simulink model "sampleModel1733_sub_sub"  (R2023a)
settings: Solver=VariableStepAuto  StartTime=0.0  StopTime=10.0  RelTol=1e-3
libraries: hdlsllib x4, simulink x1
settings Model: Creator=user1  LastModifiedBy=user1

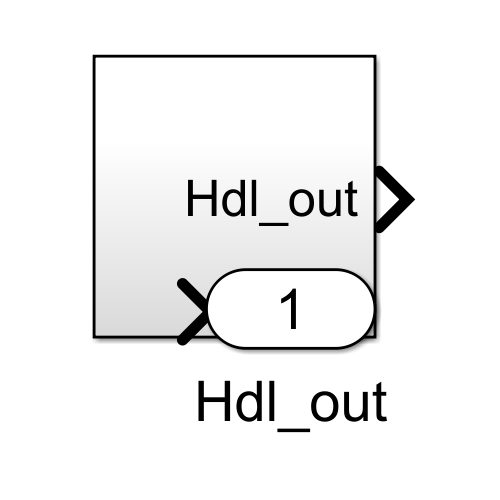
[thumbnail: Simulink's stored preview of the top-level diagram]
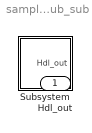
== system sampleModel1733_sub_sub ==
  Subsystem : Subsystem
  Hdl_out : Outport  OutDataTypeStr=uint8

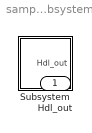
== system sampleModel1733_sub_sub/Subsystem ==
  Subsystem : Subsystem
  Hdl_out : Outport  OutDataTypeStr=uint8

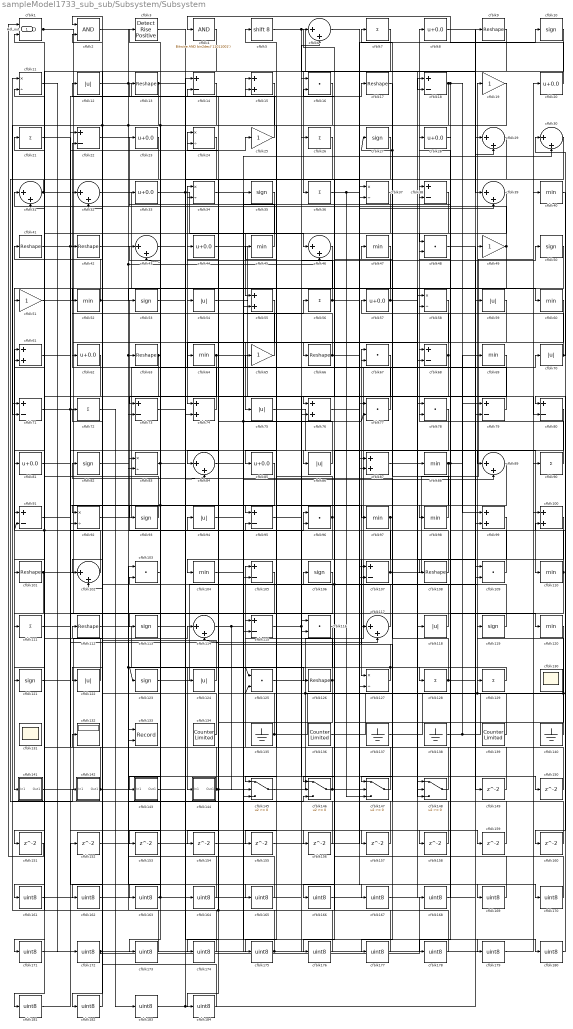
== system sampleModel1733_sub_sub/Subsystem/Subsystem ==
  cfblk1 : Logic  AllPortsSameDT=off  OutDataTypeStr=boolean
  cfblk{10,27,35,50,53,82,93,106,113,119,121,123} (12 alike) : Signum
  cfblk{15,55,61,74,76,87,99..100} (8 alike) : Sum  OutDataTypeStr=uint8
  cfblk{9,13,17,41..42,63,66,101,108,112,126} (11 alike) : Reshape
  cfblk{6,29..32,39,43,46,84,89,102,114,117} (13 alike) : Sum  Inputs=|++  OutDataTypeStr=uint8
  cfblk{16,48,67,77..78,96,103,109,116,125} (10 alike) : DotProduct  OutDataTypeStr=uint8
  cfblk{40,45,47,52,60,64,69,88,97..98,104,110,120} (13 alike) : MinMax  OutDataTypeStr=uint8
  cfblk{14,18,22,38,68,71,73,79..80,91,95,105,107,115} (14 alike) : Sum  Inputs=+-  OutDataTypeStr=uint8
  cfblk{11,24,34,37,58,83,92,127} (8 alike) : Product  Inputs=*/  OutDataTypeStr=uint8  RndMeth=Zero  SaturateOnIntegerOverflow=on
  cfblk{7,21,26,36,56,72,90,111,128..129} (10 alike) : Sum  Inputs=+  OutDataTypeStr=uint8
  cfblk{12,54,59,70,75,86,94,118,122,124} (10 alike) : Abs  OutDataTypeStr=uint8  SaturateOnIntegerOverflow=off
  cfblk130 : Scope
      settings: Floating=on
  cfblk131 : Scope
      settings: Floating=on
  cfblk132 : Display
  cfblk133 : Record  FileSettingsInternal="{\"entries\":[{\"content\":{\"excelSettings\":{\"content\":{},\"type\":\"Streamout.ExcelSettings\"}},\"type\":\"Streamout.FileSettingStorage\",\"uuid\":\"\"}],\"packageUris\":[\"http:\\/\\/schema.mathworks.com\\/mf0\\/streamout_blocks\\/R2020a\"],\"version\":\"1.0\"}"  Layout=[1 1]  SignalsInternal="{\"entries\":[{\"content\":{\"signals\":[{\"content\":{\"blockPath\":[],\"dimensions\":[1],\"domain\":\"\",\"lineColor\":\"#a2142f\",\"plots\":[1],\"port\":1,\"signalID\":38492,\"signalName\":\"cfblk175\"},\"type\":\"RecordBlkView.Signal\",\"uuid\":\"\"},{\"content\":{\"blockPath\":[],\"dimensions\":[1],\"domain\":\"\",\"lineColor\":\"#139fff\",\"plots\":[1],\"port\":2,\"signalID\":38495,\"signalName\":\"cfblk63\"},\"type\":\"RecordBlkView.Signal\",\"uuid\":\"\"}]},\"type\":\"RecordBlkView.InputSignals\",\"uuid\":\"\"}],\"packageUris\":[\"http:\\/\\/schema.mathworks.com\\/mf0\\/streamout_blocks\\/R2020a\"],\"version\":\"1.0\"}"  VisualizationBindings="{\"xyplotplugin\":{\"info\":[{\"series\":[{\"bindingParametersList\":[{\"parameter\":\"X-Axis\",\"signalID\":38492,\"signalName\":\"cfblk175\"},{\"parameter\":\"Y-Axis\",\"signalID\":38495,\"signalName\":\"cfblk63\"}],\"seriesID\":16748}],\"subplotID\":1}]}}"  CompatibilityTag=XY  st=-1
  cfblk134 : hdlsllib/Sources/Counter Limited  uplimit=7  tsamp=-1
  cfblk{135,137..138,140} (4 alike) : Ground
  cfblk136 : hdlsllib/Sources/Counter Limited  uplimit=7  tsamp=-1
  cfblk139 : hdlsllib/Sources/Counter Limited  uplimit=7  tsamp=-1
  cfblk141 : Subsystem
      settings: LibrarySourceBlock=|
      | hdlsllib/Ports &
      | Subsystems/Subsystem
  cfblk142 : Subsystem
      settings: LibrarySourceBlock=|
      | hdlsllib/Ports &
      | Subsystems/Subsystem
  cfblk143 : Subsystem
      settings: LibrarySourceBlock=|
      | hdlsllib/Ports &
      | Subsystems/Subsystem
  cfblk144 : Subsystem
      settings: LibrarySourceBlock=|
      | hdlsllib/Ports &
      | Subsystems/Subsystem
  cfblk{145..148} (4 alike) : Switch  OutDataTypeStr=uint8  SaturateOnIntegerOverflow=off  InputSameDT=off
  cfblk{149..160} (12 alike) : Delay  SampleTime=1
  cfblk{161..184} (24 alike) : DataTypeConversion  OutDataTypeStr=uint8  SaturateOnIntegerOverflow=off  RndMeth=Floor
  cfblk{19,25,49,51,65} (5 alike) : Gain  OutDataTypeStr=uint8
  cfblk2 : Logic  AllPortsSameDT=off  OutDataTypeStr=boolean
  cfblk{8,20,23,28,33,44,57,62,81,85} (10 alike) : Bias  Bias=0.0  SaturateOnIntegerOverflow=off
  cfblk3 : hdlsllib/Logic and Bit Operations/Detect Rise Positive  vinit=0  OutDataTypeStr=uint8
  cfblk4 : simulink/Logic and Bit Operations/Bitwise Operator  logicop=AND  UseBitMask=on  BitMask=bin2dec('11011001')  BitMaskRealWorld=Stored Integer
      settings: LibrarySourceBlock=|
      | hdlsllib/Logic and Bit
      | Operations/Bitwise
      | Operator
  cfblk5 : ArithShift  BitShiftNumber=8
  Hdl_out : Outport  OutDataTypeStr=uint8
  wires:
  cfblk184/1 -> cfblk72/1
  cfblk183/1 -> cfblk14/1, cfblk9/1
  cfblk182/1 -> cfblk62/1
  cfblk19/1 -> cfblk182/1
  cfblk181/1 -> cfblk152/1
  cfblk62/1 -> cfblk181/1
  cfblk180/1 -> cfblk100/2
  cfblk179/1 -> cfblk100/1
  cfblk34/1 -> cfblk179/1
  cfblk178/1 -> cfblk112/1
  cfblk100/1 -> cfblk178/1
  cfblk177/1 -> cfblk16/2
  cfblk176/1 -> cfblk16/1
  cfblk120/1 -> cfblk176/1
  cfblk175/1 -> cfblk133/1, cfblk24/2, cfblk20/1
  cfblk174/1 -> cfblk11/2
  cfblk173/1 -> cfblk11/1
  cfblk24/1 -> cfblk173/1
  cfblk172/1 -> cfblk168/1, cfblk145/3
  cfblk171/1 -> cfblk6/2
  cfblk106/1 -> cfblk171/1
  cfblk170/1 -> cfblk6/1
  cfblk61/1 -> cfblk170/1
  cfblk169/1 -> cfblk48/2
  cfblk6/1 -> cfblk169/1
  cfblk168/1 -> cfblk78/2
  cfblk167/1 -> cfblk78/1
  cfblk166/1 -> cfblk109/1
  cfblk78/1 -> cfblk166/1
  cfblk165/1 -> cfblk103/2
  cfblk153/1 -> cfblk165/1
  cfblk164/1 -> cfblk103/1
  cfblk43/1 -> cfblk164/1
  cfblk163/1 -> cfblk3/1, cfblk116/1
  cfblk162/1 -> cfblk26/1
  cfblk37/1 -> cfblk162/1
  cfblk161/1 -> cfblk35/1
  cfblk26/1 -> cfblk161/1
  cfblk160/1 -> cfblk71/1
  cfblk40/1 -> cfblk160/1
  cfblk159/1 -> cfblk117/1
  cfblk143/1(Out1) -> cfblk159/1
  cfblk158/1 -> cfblk18/1
  cfblk21/1 -> cfblk158/1
  cfblk157/1 -> cfblk31/2
  cfblk156/1 -> cfblk2/2
  cfblk155/1 -> cfblk37/1
  cfblk89/1 -> cfblk155/1
  cfblk154/1 -> cfblk146/2
  cfblk116/1 -> cfblk153/1
  cfblk152/1 -> cfblk127/2
  cfblk151/1 -> cfblk1/1
  cfblk105/1 -> cfblk151/1
  cfblk150/1 -> cfblk95/2
  cfblk84/1 -> cfblk150/1
  cfblk149/1 -> cfblk22/1
  cfblk48/1 -> cfblk149/1
  cfblk80/1 -> cfblk108/1
  cfblk45/1 -> cfblk13/1
  cfblk53/1 -> cfblk147/2
  cfblk79/1 -> cfblk64/1
  cfblk142/1(Out1) -> cfblk132/1, cfblk146/3
  cfblk18/1 -> cfblk98/1, cfblk99/1, cfblk83/2
  cfblk82/1 -> cfblk83/1
  cfblk111/1 -> cfblk117/2
  cfblk81/1 -> cfblk25/1
  cfblk137/1 -> cfblk59/1
  cfblk127/1 -> cfblk123/1, cfblk14/2
  cfblk31/1 -> cfblk142/1(In1), cfblk115/2
  cfblk63/1 -> cfblk43/1, cfblk133/2
  cfblk144/1(Out1) -> cfblk114/2, cfblk89/2, cfblk91/1
  cfblk32/1 -> cfblk68/2
  cfblk128/1 -> cfblk82/1, cfblk29/2
  cfblk86/1 -> cfblk54/1
  cfblk15/1 -> cfblk52/1, cfblk71/2, cfblk73/2, cfblk73/1
  cfblk52/1 -> cfblk1/2, cfblk60/1
  cfblk69/1 -> cfblk76/2
  cfblk95/1 -> cfblk70/1
  cfblk22/1 -> cfblk148/2
  cfblk17/1 -> cfblk147/1
  cfblk121/1 -> cfblk96/1
  cfblk76/1 -> cfblk10/1
  cfblk97/1 -> cfblk177/1, cfblk184/1
  cfblk134/1 -> cfblk32/2
  cfblk54/1 -> cfblk118/1
  cfblk71/1 -> cfblk107/2, cfblk87/2, cfblk17/1
  cfblk113/1 -> cfblk67/2
  cfblk57/1 -> cfblk31/1, cfblk109/2
  cfblk59/1 -> cfblk97/1
  cfblk39/1 -> cfblk55/1
  cfblk139/1 -> cfblk129/1
  cfblk66/1 -> cfblk24/1, cfblk39/2
  cfblk58/1 -> cfblk85/1
  cfblk83/1 -> cfblk143/1(In1), cfblk180/1
  cfblk68/1 -> cfblk47/1, cfblk174/1
  cfblk13/1 -> cfblk102/2, cfblk156/1
  cfblk91/1 -> cfblk42/1
  cfblk10/1 -> cfblk74/2
  cfblk56/1 -> cfblk34/2, cfblk89/1
  cfblk11/1 -> cfblk172/1
  cfblk93/1 -> cfblk61/2
  cfblk12/1 -> cfblk15/2, cfblk79/2
  cfblk4/1 -> cfblk101/1
  cfblk8/1 -> cfblk29/1
  cfblk27/1 -> cfblk92/1
  cfblk122/1 -> cfblk21/1, cfblk91/2
  cfblk16/1 -> cfblk175/1
  cfblk51/1 -> cfblk148/1
  cfblk72/1 -> cfblk183/1
  cfblk75/1 -> cfblk110/1
  cfblk117/1 -> cfblk5/1
  cfblk65/1 -> cfblk32/1
  cfblk85/1 -> cfblk113/1, cfblk102/1
  cfblk107/1 -> cfblk40/1, cfblk94/1
  cfblk33/1 -> cfblk46/1, cfblk84/2
  cfblk73/1 -> cfblk65/1
  cfblk118/1 -> cfblk15/1
  cfblk7/1 -> cfblk122/1
  cfblk136/1 -> cfblk119/1, cfblk90/1
  cfblk114/1 -> cfblk77/2, cfblk30/2, cfblk145/2
  cfblk124/1 -> cfblk12/1
  cfblk14/1 -> cfblk81/1, cfblk43/2
  cfblk135/1 -> cfblk107/1, cfblk44/1
  cfblk110/1 -> cfblk28/1, cfblk128/1
  cfblk29/1 -> cfblk66/1
  cfblk146/1 -> cfblk77/1, cfblk33/1
  cfblk87/1 -> cfblk88/1
  cfblk30/1 -> cfblk84/1
  cfblk5/1 -> cfblk39/1, cfblk18/2
  cfblk102/1 -> cfblk61/1
  cfblk140/1 -> cfblk49/1, cfblk125/2
  cfblk115/1 -> cfblk50/1, cfblk148/3
  cfblk98/1 -> cfblk7/1, cfblk27/1
  cfblk38/1 -> cfblk145/1
  cfblk49/1 -> cfblk23/1, cfblk55/2
  cfblk148/1 -> cfblk106/1
  cfblk99/1 -> cfblk127/1
  cfblk35/1 -> cfblk121/1
  cfblk64/1 -> cfblk116/2, cfblk92/2
  cfblk77/1 -> cfblk22/2
  cfblk2/1 -> cfblk63/1, cfblk157/1
  cfblk112/1 -> cfblk126/1
  cfblk101/1 -> cfblk111/1, cfblk124/1
  cfblk47/1 -> cfblk76/1
  cfblk50/1 -> cfblk51/1
  cfblk104/1 -> cfblk56/1
  cfblk3/1 -> cfblk37/2
  cfblk70/1 -> cfblk57/1, cfblk30/1
  cfblk9/1 -> cfblk36/1
  cfblk109/1 -> cfblk58/2
  cfblk141/1(Out1) -> cfblk114/1
  cfblk36/1 -> cfblk87/1, cfblk147/3
  cfblk41/1 -> cfblk86/1, cfblk93/1
  cfblk145/1 -> cfblk58/1, cfblk99/2
  cfblk125/1 -> cfblk67/1
  cfblk103/1 -> cfblk163/1
  cfblk28/1 -> cfblk48/1
  cfblk42/1 -> cfblk125/1, cfblk167/1, cfblk46/2
  cfblk46/1 -> cfblk141/1(In1)
  cfblk94/1 -> cfblk38/2
  cfblk60/1 -> cfblk75/1
  cfblk119/1 -> cfblk41/1, cfblk96/2
  cfblk123/1 -> cfblk19/1
  cfblk88/1 -> cfblk38/1, cfblk79/1, cfblk146/1
  cfblk44/1 -> cfblk80/2
  cfblk108/1 -> cfblk53/1
  cfblk126/1 -> cfblk115/1, cfblk154/1
  cfblk67/1 -> cfblk105/2
  cfblk147/1 -> cfblk105/1
  cfblk55/1 -> cfblk74/1
  cfblk25/1 -> cfblk2/1
  cfblk129/1 -> cfblk144/1(In1)
  cfblk74/1 -> cfblk34/1
  cfblk96/1 -> cfblk104/1, cfblk45/1
  cfblk1/1 -> cfblk95/1, Hdl_out/1
  cfblk138/1 -> cfblk80/1, cfblk69/1
  cfblk23/1 -> cfblk120/1
  cfblk92/1 -> cfblk68/1
  cfblk20/1 -> cfblk4/1
  cfblk90/1 -> cfblk8/1

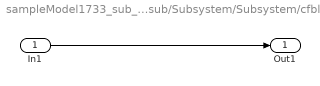
== system sampleModel1733_sub_sub/Subsystem/Subsystem/cfblk141 ==
  In1 : Inport
  Out1 : Outport
  wires:
  In1/1 -> Out1/1

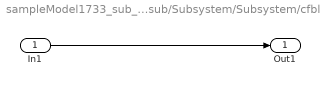
== system sampleModel1733_sub_sub/Subsystem/Subsystem/cfblk142 ==
  In1 : Inport
  Out1 : Outport
  wires:
  In1/1 -> Out1/1

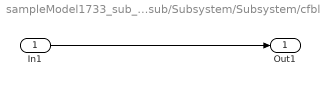
== system sampleModel1733_sub_sub/Subsystem/Subsystem/cfblk143 ==
  In1 : Inport
  Out1 : Outport
  wires:
  In1/1 -> Out1/1

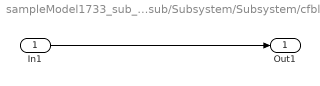
== system sampleModel1733_sub_sub/Subsystem/Subsystem/cfblk144 ==
  In1 : Inport
  Out1 : Outport
  wires:
  In1/1 -> Out1/1
